simulink library "bcm"  (R2021b)
settings: Solver=VariableStepAuto  StartTime=0.0  StopTime=10.0  RelTol=1e-3
undefined symbols (not defined in the file or in its folder): ENUM_ANTITHEFT_ALARM, ENUM_ANTITHEFT_ARM, ENUM_ANTITHEFT_DISARM, ENUM_ANTITHEFT_WAIT, ENUM_GEARPOSNTOCAN_P, ENUM_PDKEYRAWLULOCK_INUNLOCK, ENUM_PDKEYRAWPS_INPS, ENUM_POWERSTA_ON, ENUM_POWERSTA_READY, ENUM_POWERSTA_STANDBY, ENUM_PWRSTASW_ON, ENUM_PWRSTASW_READY, ENUM_VEHICLETYPE_D21, ENUM_VEHICLETYPE_D31F25, ENUM_VEHICLETYPE_D31HAWD, ENUM_VEHICLETYPE_D31HRWD, ENUM_VEHICLETYPE_D31L24, FALSE, KBCM_ACCSwcPrsTmr_s, KBCM_ALMBrightnessDark_enum, KBCM_AmbBlue_enum, KBCM_AmbBreathT_ms, KBCM_AmbGreen_enum, KBCM_AmbMidPple_enum, KBCM_AmbRed_enum, KBCM_AmbTempCtrlEN_flg, KBCM_AmbTempT_s, KBCM_AmbWelModeENWait_s, KBCM_Antitheft_enum_ovrdflg, KBCM_Antitheft_enum_ovrdval, KBCM_APMDoorCtrlSta_flg_ovrdflg, KBCM_APMDoorCtrlSta_flg_ovrdval, KBCM_CmdKeepT_s, KBCM_CSWLightRstDebT_s, KBCM_CSWTurnLPRstT_s, KBCM_DelayTSW_flg, KBCM_DiagDRLOFF_flg, KBCM_DiagFLTC_mA, KBCM_DiagFMHT_s, KBCM_DiagFRTC_mA, KBCM_DiagRLTC_mA, KBCM_DiagRRTC_mA, KBCM_DrAPMRetryTimes_cnt, KBCM_DrOpenWdwOT_s, KBCM_DrOpenWdwReady_s, KBCM_ESSOffT_ms, KBCM_ESSOnT_ms, KBCM_FDCDKCReDetectT_K, KBCM_FDCDKCUSSFilterT_K, KBCM_HandleLampKeepT_s, KBCM_IVIRstHoldT_ms, KBCM_IVIRstTriggerT_ms, KBCM_ONDelayT_ms, KBCM_RAPSAbnFlashOFFT_ms, KBCM_RAPSAbnFlashONT_ms, KBCM_ReDetectT_K, KBCM_RightHandDriveEN_flg, KBCM_RLSLowSpdFilterT_s, KBCM_RmLampKeep_min, KBCM_RmLpKeyInT_s ... (+37)
libraries: simulink x389, $bdroot x11, hcu_lib x2
(part 6 of 13)

== system bcm/BCM/BCM/PTG/KeyDetected ==
  VBCM_PASDRMR_cm : Inport
  VBCM_USSFilterT_K : Inport  Port=2
  VBCM_PASDRML_cm : Inport  Port=3
  AND{,1,3..4} (4 alike) : Logic  AllPortsSameDT=off  OutDataTypeStr=boolean
  AND2 : Logic  Inputs=3  AllPortsSameDT=off  OutDataTypeStr=boolean
  AND5 : Logic  Inputs=3  AllPortsSameDT=off  OutDataTypeStr=boolean
  Add : Sum
  Add1 : Sum  Inputs=-++
  Add2 : Sum  Inputs=--
  CheckSignalAvailable : Subsystem
  Compare To Constant2 : simulink/Logic and Bit Operations/Compare To Constant  relop=<=  const=KBCM_SPTGUpperBound_cm  OutDataTypeStr=boolean
  Compare To Constant3 : simulink/Logic and Bit Operations/Compare To Constant  relop=>=  const=KBCM_SPTGLowerBound_cm  OutDataTypeStr=boolean
  Constant : Constant  Value=KBCM_SPTGRightBound_cm
  Constant10 : Constant  Value=KBCM_USSDis_cm
  Constant11 : Constant  Value=KBCM_SPTGUpperBoundOut_cm
  Constant12 : Constant  Value=KBCM_SPTGLowerBoundOut_cm
  Constant13 : Constant  Value=KBCM_SPTGRightBoundOut_cm
  Constant15 : Constant  Value=-1  OutDataTypeStr=single
  Constant16 : Constant  Value=0  OutDataTypeStr=single
  Constant17 : Constant  Value=KBCM_SPTGUpperBound_cm
  Constant18 : Constant  Value=KBCM_SPTGLowerBound_cm
  Constant2 : Constant  Value=KBCM_SPTGLeftBound_cm
  Constant3 : Constant  Value=-1  OutDataTypeStr=single
  Constant4 : Constant  Value=KBCM_USSDis_cm
  Constant5 : Constant  Value=0  OutDataTypeStr=single
  Constant6 : Constant  Value=KBCM_SPTGLeftBoundOut_cm
  Constant7 : Constant  Value=KBCM_USSDis_cm
  Constant8 : Constant  Value=KBCM_SPTGLeftBound_cm
  Constant9 : Constant  Value=KBCM_SPTGLeftBound_cm
  Data Type Conversion : DataTypeConversion  OutDataTypeStr=single
  Data Type Conversion1 : DataTypeConversion  OutDataTypeStr=single
  Data Type Conversion2 : DataTypeConversion  OutDataTypeStr=boolean
  Data Type Conversion3 : DataTypeConversion  OutDataTypeStr=boolean
  Detect Decrease : simulink/Logic and Bit Operations/Detect Decrease  vinit=0.0  OutDataTypeStr=boolean
  Detect Decrease1 : simulink/Logic and Bit Operations/Detect Decrease  vinit=0.0  OutDataTypeStr=boolean
  Equal : RelationalOperator  OutDataTypeStr=boolean  RndMeth=Simplest
  Gain : Gain  Gain=-1
  GreaterThan : RelationalOperator  Operator=<=  OutDataTypeStr=boolean  RndMeth=Simplest
  GreaterThan1 : RelationalOperator  Operator=<=  OutDataTypeStr=boolean  RndMeth=Simplest
  GreaterThan2 : RelationalOperator  OutDataTypeStr=boolean  RndMeth=Simplest
  Less Than : RelationalOperator  Operator=<=  OutDataTypeStr=boolean  RndMeth=Simplest
  Less Than1 : RelationalOperator  OutDataTypeStr=boolean  RndMeth=Simplest
  Product : Product
  Sum1 : Sum
  Sum2 : Sum  Inputs=|++
  Sum3 : Sum  Inputs=|+-
  Sum4 : Sum
  Switch{1..6} (6 alike) : Switch  Criteria=u2 > Threshold
  Target_h : Subsystem
  Unit Delay{1..6} (6 alike) : UnitDelay  SampleTime=-1  HasFrameUpgradeWarning=on
  cosRML : Subsystem
  KeyDetected : Outport
  KeyDetectedOut : Outport  Port=2
  wires:
  Constant4/1 -> CheckSignalAvailable/3(KBCM_USSDis_cm_IN)
  CheckSignalAvailable/1(VBCM_PASDRML_cm) -> cosRML/1(VBCM_PASDRML_cm), Target_h/1(VBCM_PASDRML_cm), Product/2
  CheckSignalAvailable/2(VBCM_PASDRMR_cm) -> Target_h/2(VBCM_PASDRMR_cm), cosRML/2(VBCM_PASDRMR_cm)
  CheckSignalAvailable/3(KBCM_USSDis_cm) -> Target_h/3(KBCM_USSDis_cm), cosRML/3(KBCM_USSDis_cm)
  Target_h/1(Target_h) -> Compare To Constant2/1, Compare To Constant3/1, Less Than/1, Less Than1/1
  Compare To Constant2/1 -> AND1/1
  Compare To Constant3/1 -> AND1/2
  AND1/1 -> AND2/2
  AND/1 -> AND2/1
  cosRML/1(cosRML) -> Product/1
  CheckSignalAvailable/4(CheckResult) -> [CheckResult]
  [CheckResult] -> AND2/3
  Detect Decrease/1 -> Switch2/2
  Switch2/1 -> Data Type Conversion/1
  Sum1/1 -> Switch2/3
  Unit Delay2/1 -> Switch3/2, Sum1/2, Switch4/2
  Constant3/1 -> Switch3/1
  Constant5/1 -> Switch3/3
  Switch3/1 -> Sum1/1
  Switch4/1 -> Data Type Conversion2/1, KeyDetected/1
  Unit Delay4/1 -> Switch4/1
  VBCM_PASDRML_cm/1 -> CheckSignalAvailable/1(VBCM_PASDRML_cm_IN)
  VBCM_PASDRMR_cm/1 -> CheckSignalAvailable/2(VBCM_PASDRMR_cm_IN)
  AND2/1 -> Unit Delay6/1, Detect Decrease/1
  GreaterThan1/1 -> AND4/1
  Add1/1 -> GreaterThan1/2
  [Target_x] -> GreaterThan1/1, GreaterThan2/1
  Product/1 -> [Target_x]
  [Target_x] -> Equal/1, GreaterThan/1
  Constant17/1 -> Sum2/1
  Constant11/1 -> Sum2/2
  Constant12/1 -> Sum3/2
  Constant18/1 -> Sum3/1
  [CheckResult] -> AND5/3
  AND3/1 -> AND5/1
  AND4/1 -> AND5/2
  AND5/1 -> Unit Delay1/1, Detect Decrease1/1
  Unit Delay5/1 -> Switch6/1
  Switch6/1 -> KeyDetectedOut/1, Data Type Conversion3/1
  Switch5/1 -> Sum4/1
  Constant16/1 -> Switch5/3
  Constant15/1 -> Switch5/1
  Unit Delay3/1 -> Switch6/2, Sum4/2, Switch5/2
  Sum4/1 -> Switch1/3
  Switch1/1 -> Data Type Conversion1/1
  Detect Decrease1/1 -> Switch1/2
  Sum2/1 -> Less Than/2
  Less Than/1 -> AND3/1
  Sum3/1 -> Less Than1/2
  Less Than1/1 -> AND3/2
  Constant10/1 -> Add1/2
  Constant9/1 -> Add1/1
  Constant13/1 -> Add1/3
  Constant7/1 -> Add/2
  Equal/1 -> AND/1
  GreaterThan/1 -> AND/2
  Constant/1 -> Add/1
  Add/1 -> GreaterThan/2
  GreaterThan2/1 -> AND4/2
  Constant2/1 -> Add2/1
  Constant6/1 -> Add2/2
  Add2/1 -> GreaterThan2/2
  Unit Delay1/1 -> Switch6/3
  Unit Delay6/1 -> Switch4/3
  Constant8/1 -> Gain/1
  Gain/1 -> Equal/2
  Data Type Conversion/1 -> Unit Delay2/1
  Data Type Conversion1/1 -> Unit Delay3/1
  Data Type Conversion2/1 -> Unit Delay4/1
  Data Type Conversion3/1 -> Unit Delay5/1
  VBCM_USSFilterT_K/1 -> [VBCM_USSFilterT_K]
  [VBCM_USSFilterT_K] -> Switch2/1
  [VBCM_USSFilterT_K] -> Switch1/1

== system bcm/BCM/BCM/PTG/Subsystem1 ==
  VAPM_PASDRMR_cm : Inport
  Add4 : Sum
  Compare To Constant1 : simulink/Logic and Bit Operations/Compare To Constant  relop=~=  const=0  OutDataTypeStr=boolean
  Compare To Constant6 : simulink/Logic and Bit Operations/Compare To Constant  relop===  const=0  OutDataTypeStr=boolean
  Compare To Constant8 : simulink/Logic and Bit Operations/Compare To Constant  relop===  const=255  OutDataTypeStr=boolean
  Constant1 : Constant  Value=0  OutDataTypeStr=uint8
  Constant12 : Constant  OutDataTypeStr=uint8
  Constant13 : Constant  Value=0  OutDataTypeStr=uint8
  Constant2 : Constant  OutDataTypeStr=uint8
  Constant3 : Constant  Value=KBCM_SPTGTOut_K
  Constant4 : Constant  Value=255  OutDataTypeStr=uint8
  Constant5 : Constant  Value=KBCM_SPTGTOut_K
  Detect Change : simulink/Logic and Bit Operations/Detect Change  vinit=0  OutDataTypeStr=boolean
  Equal : RelationalOperator  OutDataTypeStr=boolean  RndMeth=Simplest
  Equal1 : RelationalOperator  Operator===  OutDataTypeStr=boolean  RndMeth=Simplest
  Equal2 : RelationalOperator  Operator=~=  OutDataTypeStr=boolean  RndMeth=Simplest
  Logical Operator : Logic  Inputs=3  AllPortsSameDT=off  OutDataTypeStr=boolean
  Logical Operator2 : Logic  Operator=OR  AllPortsSameDT=off  OutDataTypeStr=boolean
  Switch{2..3,8..9} (4 alike) : Switch  Criteria=u2 > Threshold
  Unit Delay2 : UnitDelay  SampleTime=-1  HasFrameUpgradeWarning=on
  Unit Delay6 : UnitDelay  SampleTime=-1  HasFrameUpgradeWarning=on
  PASDRMR : Outport
  wires:
  Equal1/1 -> Logical Operator2/2
  Switch9/1 -> Add4/1
  Constant5/1 -> Equal2/2, Equal1/1
  Unit Delay6/1 -> Equal/1, Add4/2
  Compare To Constant8/1 -> Switch8/2
  Equal2/1 -> Logical Operator2/1
  Constant4/1 -> Switch3/3
  Switch2/1 -> Unit Delay2/1, Switch3/1
  Compare To Constant1/1 -> Logical Operator/2
  Logical Operator/1 -> Switch2/2
  Constant13/1 -> Switch9/1
  Add4/1 -> Switch8/1
  Unit Delay2/1 -> Switch2/3
  Constant12/1 -> Switch9/3
  Equal/1 -> Switch9/2
  Constant3/1 -> Equal/2
  Detect Change/1 -> Logical Operator/1
  Compare To Constant6/1 -> Logical Operator/3
  Constant1/1 -> Switch8/3
  Switch3/1 -> PASDRMR/1
  VAPM_PASDRMR_cm/1 -> Switch2/1, Detect Change/1, Compare To Constant1/1, Compare To Constant8/1
  Logical Operator2/1 -> Switch3/2
  Constant2/1 -> Equal1/2
  Switch8/1 -> Unit Delay6/1, Compare To Constant6/1, Equal2/1

== system bcm/BCM/BCM/PTG/Subsystem3 ==
  VAPM_PASDRML_cm : Inport
  Add4 : Sum
  Compare To Constant1 : simulink/Logic and Bit Operations/Compare To Constant  relop=~=  const=0  OutDataTypeStr=boolean
  Compare To Constant6 : simulink/Logic and Bit Operations/Compare To Constant  relop===  const=0  OutDataTypeStr=boolean
  Compare To Constant8 : simulink/Logic and Bit Operations/Compare To Constant  relop===  const=255  OutDataTypeStr=boolean
  Constant1 : Constant  Value=0  OutDataTypeStr=uint8
  Constant12 : Constant  OutDataTypeStr=uint8
  Constant13 : Constant  Value=0  OutDataTypeStr=uint8
  Constant2 : Constant  Value=0  OutDataTypeStr=uint8
  Constant3 : Constant  Value=KBCM_SPTGTOut_K
  Constant4 : Constant  Value=255  OutDataTypeStr=uint8
  Constant5 : Constant  Value=KBCM_SPTGTOut_K
  Detect Change : simulink/Logic and Bit Operations/Detect Change  vinit=0  OutDataTypeStr=boolean
  Equal : RelationalOperator  OutDataTypeStr=boolean  RndMeth=Simplest
  Equal1 : RelationalOperator  Operator===  OutDataTypeStr=boolean  RndMeth=Simplest
  Equal2 : RelationalOperator  Operator=~=  OutDataTypeStr=boolean  RndMeth=Simplest
  Logical Operator : Logic  Inputs=3  AllPortsSameDT=off  OutDataTypeStr=boolean
  Logical Operator2 : Logic  Operator=OR  AllPortsSameDT=off  OutDataTypeStr=boolean
  Switch{2..3,8..9} (4 alike) : Switch  Criteria=u2 > Threshold
  Unit Delay2 : UnitDelay  SampleTime=-1  HasFrameUpgradeWarning=on
  Unit Delay6 : UnitDelay  SampleTime=-1  HasFrameUpgradeWarning=on
  PASDRML : Outport
  wires:
  Constant2/1 -> Equal1/2
  Logical Operator2/1 -> Switch3/2
  VAPM_PASDRML_cm/1 -> Switch2/1, Detect Change/1, Compare To Constant1/1, Compare To Constant8/1
  Switch3/1 -> PASDRML/1
  Constant1/1 -> Switch8/3
  Compare To Constant6/1 -> Logical Operator/3
  Detect Change/1 -> Logical Operator/1
  Constant3/1 -> Equal/2
  Equal/1 -> Switch9/2
  Constant12/1 -> Switch9/3
  Unit Delay2/1 -> Switch2/3
  Add4/1 -> Switch8/1
  Constant13/1 -> Switch9/1
  Switch8/1 -> Equal2/1, Compare To Constant6/1, Unit Delay6/1
  Logical Operator/1 -> Switch2/2
  Compare To Constant1/1 -> Logical Operator/2
  Switch2/1 -> Unit Delay2/1, Switch3/1
  Constant4/1 -> Switch3/3
  Equal2/1 -> Logical Operator2/1
  Compare To Constant8/1 -> Switch8/2
  Unit Delay6/1 -> Equal/1, Add4/2
  Constant5/1 -> Equal2/2, Equal1/1
  Switch9/1 -> Add4/1
  Equal1/1 -> Logical Operator2/2

== system bcm/BCM/BCM/Personal_Setting/ACC ==
  UserNow : Inport
  Loadbar : Inport  Port=2
  UpdateReq : Inport  Port=3
  task_time_s : Inport  Port=4
  VINP_TimeGapLevel_enum : Inport  Port=5
  VINP_FlashACCLevelSta12_enum : Inport  Port=6
  VINP_FlashACCLevelSta34_enum : Inport  Port=7
  VINP_FlashACCLevelSta57_enum : Inport  Port=8
  VINP_SWC2LRightSta_flg : Inport  Port=9
  VINP_SWC2LLeftSta_flg : Inport  Port=10
  VINP_FDCVMCSpdCtrlModeSta_enum : Inport  Port=11
  VINP_ADASACCSta_enum : Inport  Port=12
  VINP_VehicleType_enum : Inport  Port=13
  AND : Logic  Inputs=3  AllPortsSameDT=off  OutDataTypeStr=boolean
  AND1 : Logic  AllPortsSameDT=off  OutDataTypeStr=boolean
  AND2 : Logic  AllPortsSameDT=off  OutDataTypeStr=boolean
  AND3 : Logic  AllPortsSameDT=off  OutDataTypeStr=boolean
  Chart : Stateflow chart  TreatAsAtomicUnit=on
  Compare To Constant : simulink/Logic and Bit Operations/Compare To Constant  relop===  const=1  OutDataTypeStr=boolean
  Compare To Constant1 : simulink/Logic and Bit Operations/Compare To Constant  relop=~=  const=0  OutDataTypeStr=boolean
  Compare To Constant2 : simulink/Logic and Bit Operations/Compare To Constant  relop=~=  const=5  OutDataTypeStr=boolean
  Compare To Constant3 : simulink/Logic and Bit Operations/Compare To Constant  relop=~=  const=6  OutDataTypeStr=boolean
  Constant : Constant  Value=4
  Constant1 : Constant  Value=KBCM_ACCSwcPrsTmr_s
  Constant3 : Constant  Value=KBCM_WaitACCChange_s
  Constant4 : Constant  Value=ENUM_VEHICLETYPE_D31L24
  Constant5 : Constant  Value=ENUM_VEHICLETYPE_D21
  Constant6 : Constant  Value=TRUE
  Constant7 : Constant  Value=FALSE
  Data Type Conversion : DataTypeConversion  OutDataTypeStr=uint8
  Divide : Product  Inputs=*/
  Divide1 : Product  Inputs=*/
  Equal : RelationalOperator  Operator===  OutDataTypeStr=boolean  RndMeth=Simplest
  Equal1 : RelationalOperator  Operator===  OutDataTypeStr=boolean  RndMeth=Simplest
  Logical Operator : Logic  Operator=OR  AllPortsSameDT=off  OutDataTypeStr=boolean
  Switch : Switch  Criteria=u2 ~= 0
  Switch1 : Switch  Criteria=u2 ~= 0
  Switch2 : Switch  Criteria=u2 ~= 0
  Switch3 : Switch  Criteria=u2 > Threshold
  VALUE_TYPE_ACC : Subsystem
  VBCM_TimeGapLevelSta_enum : Outport
  VBCM_ACCLevelMem12_enum : Outport  Port=2
  VBCM_ACCLevelMem34_enum : Outport  Port=3
  VBCM_ACCLevelMem57_enum : Outport  Port=4
  VBCM_LRightStaCmd_flg : Outport  Port=5
  VBCM_LLeftStaCmd_flg : Outport  Port=6
  wires:
  [task_time_s] -> Divide1/2
  Divide1/1 -> Chart/7(KBCM_WaitACCChange_s)
  Constant3/1 -> Divide1/1
  [task_time_s] -> Divide/2
  task_time_s/1 -> [task_time_s]
  Chart/2(VBCM_LLeftStaCmd_flg) -> Switch1/1
  Chart/1(VBCM_LRightStaCmd_flg) -> Switch/1
  [VINP_TimeGapLevel_enum] -> Switch2/3
  [VINP_TimeGapLevel_enum] -> Chart/2(VINP_TimeGapLevel_enum)
  VINP_TimeGapLevel_enum/1 -> [VINP_TimeGapLevel_enum]
  VALUE_TYPE_ACC/1(Setting) -> Switch2/1  "VBCM_TimeGapLevelSta_enum"
  Switch2/1 -> VBCM_TimeGapLevelSta_enum/1, [VBCM_TimeGapLevelSta_enum]  "VBCM_TimeGapLevelSta_enum"
  [VBCM_ACCUserSettingEN_flg] -> Switch2/2
  Switch1/1 -> VBCM_LLeftStaCmd_flg/1  "VBCM_LLeftStaCmd_flg"
  [VINP_SWC2LLeftSta_flg] -> Switch1/3
  [VBCM_ACCUserSettingEN_flg] -> Switch1/2
  [VINP_SWC2LRightSta_flg] -> Switch/3
  Switch/1 -> VBCM_LRightStaCmd_flg/1  "VBCM_LRightStaCmd_flg"
  [VBCM_ACCUserSettingEN_flg] -> Switch/2
  [VINP_SWC2LLeftSta_flg] -> Chart/5(VINP_SWC2LLeftSta_flg)
  [VINP_SWC2LRightSta_flg] -> Chart/4(VINP_SWC2LRightSta_flg)
  [VINP_SWC2LLeftSta_flg] -> AND3/2
  [VINP_SWC2LRightSta_flg] -> AND2/2
  VINP_SWC2LLeftSta_flg/1 -> [VINP_SWC2LLeftSta_flg]
  VINP_SWC2LRightSta_flg/1 -> [VINP_SWC2LRightSta_flg]
  Constant1/1 -> Divide/1
  Divide/1 -> Chart/6(KBCM_ACCSwcPrsTmr_s)
  [VBCM_TimeGapLevelSta_enum] -> Chart/3(VBCM_TimeGapLevelSta_enum)
  [UserNow] -> VALUE_TYPE_ACC/1(UserNow)
  UserNow/1 -> [UserNow]
  [VBCM_ACCChangeEnable_flg] -> Chart/1(VBCM_ACCChangeEnable_flg)
  [VBCM_ACCChangeEnable_flg] -> AND3/1
  [VBCM_ACCChangeEnable_flg] -> AND2/1
  AND3/1 -> VALUE_TYPE_ACC/5(MinusCmd)
  AND2/1 -> VALUE_TYPE_ACC/4(PlusCmd)
  AND1/1 -> [VBCM_ACCChangeEnable_flg]
  AND/1 -> AND1/2
  Compare To Constant/1 -> AND1/1
  VINP_ADASACCSta_enum/1 -> Compare To Constant1/1, Compare To Constant2/1, Compare To Constant3/1
  Compare To Constant3/1 -> AND/3
  Compare To Constant2/1 -> AND/2
  Compare To Constant1/1 -> AND/1
  VINP_FDCVMCSpdCtrlModeSta_enum/1 -> Compare To Constant/1
  VINP_FlashACCLevelSta12_enum/1 -> VALUE_TYPE_ACC/6(EEP_Set12)
  VINP_FlashACCLevelSta34_enum/1 -> VALUE_TYPE_ACC/7(EEP_Set34)
  VINP_FlashACCLevelSta57_enum/1 -> VALUE_TYPE_ACC/8(EEP_Set57)
  VALUE_TYPE_ACC/2(Set12) -> VBCM_ACCLevelMem12_enum/1  "VBCM_ACCLevelMem12_enum"
  VALUE_TYPE_ACC/3(Set34) -> VBCM_ACCLevelMem34_enum/1  "VBCM_ACCLevelMem34_enum"
  VALUE_TYPE_ACC/4(Set57) -> VBCM_ACCLevelMem57_enum/1  "VBCM_ACCLevelMem57_enum"
  Loadbar/1 -> VALUE_TYPE_ACC/2(Loadbar)
  UpdateReq/1 -> VALUE_TYPE_ACC/3(UpdateReq)
  Constant/1 -> Data Type Conversion/1
  Data Type Conversion/1 -> VALUE_TYPE_ACC/9(Default)
  VINP_VehicleType_enum/1 -> [VINP_VehicleType_enum]
  [VINP_VehicleType_enum] -> Equal/1
  Constant4/1 -> Equal/2
  Constant5/1 -> Equal1/2
  [VINP_VehicleType_enum] -> Equal1/1
  Equal/1 -> Logical Operator/1
  Equal1/1 -> Logical Operator/2
  Logical Operator/1 -> Switch3/2
  Constant7/1 -> Switch3/1
  Constant6/1 -> Switch3/3
  Switch3/1 -> [VBCM_ACCUserSettingEN_flg]

== system bcm/BCM/BCM/Personal_Setting/AmbLight ==
  UserNow : Inport
  Loadbar : Inport  Port=2
  VINP_CANMsgValidIVI1_flg : Inport  Port=3
  VINP_AmbLightSW_flg : Inport  Port=4
  VINP_FlashAmbFunEN_enum : Inport  Port=5
  VINP_AmbLightWlcmLightSW_flg : Inport  Port=6
  VINP_FlashAmbWelEN_enum : Inport  Port=7
  VINP_AmbLightDimInDarkSW_flg : Inport  Port=8
  VINP_FlashAmbDimEN_enum : Inport  Port=9
  VINP_LINKtoDRIVE_flg : Inport  Port=10
  VINP_FlashAmbLinkDriSta_enum : Inport  Port=11
  VINP_AmbLighLowBatAlertSW_flg : Inport  Port=12
  VINP_FlashAmbPwrWarnEN_enum : Inport  Port=13
  VINP_AmbLighSafetyAlertSW_flg : Inport  Port=14
  VINP_FlashAmbODAEN_enum : Inport  Port=15
  VINP_AmbLightColorSet_enum : Inport  Port=16
  VINP_FlashAmbColorSta1_enum : Inport  Port=17
  VINP_FlashAmbColorSta2_enum : Inport  Port=18
  VINP_FlashAmbColorSta3_enum : Inport  Port=19
  VINP_FlashAmbColorSta4_enum : Inport  Port=20
  VINP_FlashAmbColorSta5_enum : Inport  Port=21
  VINP_FlashAmbColorSta7_enum : Inport  Port=22
  VINP_AmbLightBrightnessSet_enum : Inport  Port=23
  VINP_FlashAmbBrightnessSta1_enum : Inport  Port=24
  VINP_FlashAmbBrightnessSta2_enum : Inport  Port=25
  VINP_FlashAmbBrightnessSta3_enum : Inport  Port=26
  VINP_FlashAmbBrightnessSta4_enum : Inport  Port=27
  VINP_FlashAmbBrightnessSta5_enum : Inport  Port=28
  VINP_FlashAmbBrightnessSta7_enum : Inport  Port=29
  Constant{,3..7} (6 alike) : Constant  OutDataTypeStr=boolean
  Constant1 : Constant  Value=28  OutDataTypeStr=uint8
  Constant10 : Constant  Value=101  OutDataTypeStr=uint8
  Constant2 : Constant  Value=50  OutDataTypeStr=uint8
  Constant9 : Constant  Value=64  OutDataTypeStr=uint8
  Data Type Conversion : DataTypeConversion  OutDataTypeStr=uint8
  Ground : Ground
  TOGGLE_TYPE_AmbDimEN : Subsystem
  TOGGLE_TYPE_AmbFunEN : Subsystem
  TOGGLE_TYPE_AmbLinkDriSta : Subsystem
  TOGGLE_TYPE_AmbODAEN : Subsystem
  TOGGLE_TYPE_AmbPwrWarnEN : Subsystem
  TOGGLE_TYPE_AmbWelEN : Subsystem
  VALUE_TYPE_AmbBrightnessSta : Subsystem
  VALUE_TYPE_AmbColorSta : Subsystem
  VBCM_UserNow_enum : Outport
  FDC_BCM_AmbFunEN_Sta : Outport  Port=2
  VBCM_AmbFunENMem_enum : Outport  Port=3
  FDC_BCM_AmbWelEN_Sta : Outport  Port=4
  VBCM_AmbWelENMem_enum : Outport  Port=5
  FDC_BCM_AmbDimEN_Sta : Outport  Port=6
  VBCM_AmbDimENMem_enum : Outport  Port=7
  FDC_BCM_AmbLinkDriSta_Sta : Outport  Port=8
  VBCM_AmbLinkDriStaMem_enum : Outport  Port=9
  FDC_BCM_AmbPwrWarnEN_Sta : Outport  Port=10
  VBCM_AmbPwrWarnENMem_enum : Outport  Port=11
  FDC_BCM_AmbODAEN_Sta : Outport  Port=12
  VBCM_AmbODAENMem_enum : Outport  Port=13
  FDC_BCM_AmbColorSta_Sta : Outport  Port=14
  VBCM_AmbColorSta1_enum : Outport  Port=15
  VBCM_AmbColorSta2_enum : Outport  Port=16
  VBCM_AmbColorSta3_enum : Outport  Port=17
  VBCM_AmbColorSta4_enum : Outport  Port=18
  VBCM_AmbColorSta5_enum : Outport  Port=19
  VBCM_AmbColorSta7_enum : Outport  Port=20
  FDC_BCM_AmbBrightSta_Sta : Outport  Port=21  OutDataTypeStr=uint8
  VBCM_AmbBrightnessSta1_enum : Outport  Port=22  OutDataTypeStr=uint8
  VBCM_AmbBrightnessSta2_enum : Outport  Port=23
  VBCM_AmbBrightnessSta3_enum : Outport  Port=24
  VBCM_AmbBrightnessSta4_enum : Outport  Port=25
  VBCM_AmbBrightnessSta5_enum : Outport  Port=26
  VBCM_AmbBrightnessSta7_enum : Outport  Port=27
  wires:
  VALUE_TYPE_AmbBrightnessSta/3(Set2) -> VBCM_AmbBrightnessSta2_enum/1
  VALUE_TYPE_AmbBrightnessSta/2(Set1) -> VBCM_AmbBrightnessSta1_enum/1
  [UserNow] -> VALUE_TYPE_AmbBrightnessSta/1(UserNow)
  VALUE_TYPE_AmbBrightnessSta/1(Setting) -> FDC_BCM_AmbBrightSta_Sta/1
  TOGGLE_TYPE_AmbFunEN/1(Setting) -> FDC_BCM_AmbFunEN_Sta/1
  [Loadbar] -> VALUE_TYPE_AmbColorSta/2(Loadbar)
  VALUE_TYPE_AmbBrightnessSta/6(Set5) -> VBCM_AmbBrightnessSta5_enum/1
  TOGGLE_TYPE_AmbFunEN/2(Set) -> VBCM_AmbFunENMem_enum/1
  VALUE_TYPE_AmbBrightnessSta/7(Set7) -> VBCM_AmbBrightnessSta7_enum/1
  VALUE_TYPE_AmbBrightnessSta/4(Set3) -> VBCM_AmbBrightnessSta3_enum/1
  [UserNow] -> VALUE_TYPE_AmbColorSta/1(UserNow)
  VALUE_TYPE_AmbBrightnessSta/5(Set4) -> VBCM_AmbBrightnessSta4_enum/1
  [Loadbar] -> VALUE_TYPE_AmbBrightnessSta/2(Loadbar)
  UserNow/1 -> [UserNow]
  Loadbar/1 -> [Loadbar]
  VALUE_TYPE_AmbColorSta/1(Setting) -> FDC_BCM_AmbColorSta_Sta/1
  VALUE_TYPE_AmbColorSta/2(Set1) -> VBCM_AmbColorSta1_enum/1
  VALUE_TYPE_AmbColorSta/3(Set2) -> VBCM_AmbColorSta2_enum/1
  VALUE_TYPE_AmbColorSta/4(Set3) -> VBCM_AmbColorSta3_enum/1
  VALUE_TYPE_AmbColorSta/5(Set4) -> VBCM_AmbColorSta4_enum/1
  VALUE_TYPE_AmbColorSta/6(Set5) -> VBCM_AmbColorSta5_enum/1
  VALUE_TYPE_AmbColorSta/7(Set7) -> VBCM_AmbColorSta7_enum/1
  [UserNow] -> TOGGLE_TYPE_AmbFunEN/1(UserNow)
  [Loadbar] -> TOGGLE_TYPE_AmbFunEN/2(Loadbar)
  VINP_AmbLightSW_flg/1 -> TOGGLE_TYPE_AmbFunEN/3(iviCMD)
  VINP_FlashAmbFunEN_enum/1 -> TOGGLE_TYPE_AmbFunEN/4(EEP_Set)
  Constant/1 -> TOGGLE_TYPE_AmbFunEN/5(Default)
  Constant9/1 -> VALUE_TYPE_AmbColorSta/11(NoReqV)
  Constant1/1 -> VALUE_TYPE_AmbColorSta/12(Default)
  VINP_FlashAmbColorSta7_enum/1 -> VALUE_TYPE_AmbColorSta/9(EEP_Set7)
  VINP_FlashAmbColorSta5_enum/1 -> VALUE_TYPE_AmbColorSta/8(EEP_Set5)
  VINP_FlashAmbColorSta4_enum/1 -> VALUE_TYPE_AmbColorSta/7(EEP_Set4)
  VINP_FlashAmbColorSta3_enum/1 -> VALUE_TYPE_AmbColorSta/6(EEP_Set3)
  VINP_FlashAmbColorSta2_enum/1 -> VALUE_TYPE_AmbColorSta/5(EEP_Set2)
  VINP_FlashAmbColorSta1_enum/1 -> VALUE_TYPE_AmbColorSta/4(EEP_Set1)
  Constant10/1 -> VALUE_TYPE_AmbBrightnessSta/11(NoReqV)
  Constant2/1 -> VALUE_TYPE_AmbBrightnessSta/12(Default)
  VINP_FlashAmbBrightnessSta7_enum/1 -> VALUE_TYPE_AmbBrightnessSta/9(EEP_Set7)
  VINP_FlashAmbBrightnessSta5_enum/1 -> VALUE_TYPE_AmbBrightnessSta/8(EEP_Set5)
  VINP_FlashAmbBrightnessSta4_enum/1 -> VALUE_TYPE_AmbBrightnessSta/7(EEP_Set4)
  VINP_FlashAmbBrightnessSta3_enum/1 -> VALUE_TYPE_AmbBrightnessSta/6(EEP_Set3)
  VINP_FlashAmbBrightnessSta2_enum/1 -> VALUE_TYPE_AmbBrightnessSta/5(EEP_Set2)
  VINP_FlashAmbBrightnessSta1_enum/1 -> VALUE_TYPE_AmbBrightnessSta/4(EEP_Set1)
  VINP_AmbLightBrightnessSet_enum/1 -> VALUE_TYPE_AmbBrightnessSta/3(iviCMD)
  [UserNow] -> TOGGLE_TYPE_AmbWelEN/1(UserNow)
  [Loadbar] -> TOGGLE_TYPE_AmbWelEN/2(Loadbar)
  Constant3/1 -> TOGGLE_TYPE_AmbWelEN/5(Default)
  VINP_AmbLightWlcmLightSW_flg/1 -> TOGGLE_TYPE_AmbWelEN/3(iviCMD)
  VINP_FlashAmbWelEN_enum/1 -> TOGGLE_TYPE_AmbWelEN/4(EEP_Set)
  TOGGLE_TYPE_AmbWelEN/1(Setting) -> FDC_BCM_AmbWelEN_Sta/1
  TOGGLE_TYPE_AmbWelEN/2(Set) -> VBCM_AmbWelENMem_enum/1
  [UserNow] -> TOGGLE_TYPE_AmbDimEN/1(UserNow)
  Constant4/1 -> TOGGLE_TYPE_AmbDimEN/5(Default)
  [Loadbar] -> TOGGLE_TYPE_AmbDimEN/2(Loadbar)
  VINP_AmbLightDimInDarkSW_flg/1 -> TOGGLE_TYPE_AmbDimEN/3(iviCMD)
  VINP_FlashAmbDimEN_enum/1 -> TOGGLE_TYPE_AmbDimEN/4(EEP_Set)
  TOGGLE_TYPE_AmbDimEN/1(Setting) -> FDC_BCM_AmbDimEN_Sta/1
  TOGGLE_TYPE_AmbDimEN/2(Set) -> VBCM_AmbDimENMem_enum/1
  [UserNow] -> TOGGLE_TYPE_AmbLinkDriSta/1(UserNow)
  Constant5/1 -> TOGGLE_TYPE_AmbLinkDriSta/8(Default)
  [Loadbar] -> TOGGLE_TYPE_AmbLinkDriSta/2(Loadbar)
  VINP_LINKtoDRIVE_flg/1 -> TOGGLE_TYPE_AmbLinkDriSta/6(iviCMD)
  VINP_FlashAmbLinkDriSta_enum/1 -> TOGGLE_TYPE_AmbLinkDriSta/7(EEP_Set)
  TOGGLE_TYPE_AmbLinkDriSta/1(Setting) -> FDC_BCM_AmbLinkDriSta_Sta/1
  TOGGLE_TYPE_AmbLinkDriSta/2(Set) -> VBCM_AmbLinkDriStaMem_enum/1
  Constant6/1 -> TOGGLE_TYPE_AmbPwrWarnEN/5(Default)
  [UserNow] -> TOGGLE_TYPE_AmbPwrWarnEN/1(UserNow)
  [Loadbar] -> TOGGLE_TYPE_AmbPwrWarnEN/2(Loadbar)
  VINP_AmbLighLowBatAlertSW_flg/1 -> TOGGLE_TYPE_AmbPwrWarnEN/3(iviCMD)
  VINP_FlashAmbPwrWarnEN_enum/1 -> TOGGLE_TYPE_AmbPwrWarnEN/4(EEP_Set)
  TOGGLE_TYPE_AmbPwrWarnEN/1(Setting) -> FDC_BCM_AmbPwrWarnEN_Sta/1
  TOGGLE_TYPE_AmbPwrWarnEN/2(Set) -> VBCM_AmbPwrWarnENMem_enum/1
  [UserNow] -> TOGGLE_TYPE_AmbODAEN/1(UserNow)
  [Loadbar] -> TOGGLE_TYPE_AmbODAEN/2(Loadbar)
  Constant7/1 -> TOGGLE_TYPE_AmbODAEN/5(Default)
  VINP_AmbLighSafetyAlertSW_flg/1 -> TOGGLE_TYPE_AmbODAEN/3(iviCMD)
  VINP_FlashAmbODAEN_enum/1 -> TOGGLE_TYPE_AmbODAEN/4(EEP_Set)
  TOGGLE_TYPE_AmbODAEN/1(Setting) -> FDC_BCM_AmbODAEN_Sta/1
  TOGGLE_TYPE_AmbODAEN/2(Set) -> VBCM_AmbODAENMem_enum/1
  VINP_CANMsgValidIVI1_flg/1 -> [VINP_CANMsgValidIVI1_flg]
  [VINP_CANMsgValidIVI1_flg] -> VALUE_TYPE_AmbColorSta/10(VINP_CANMsgValidIVI1_flg)
  [VINP_CANMsgValidIVI1_flg] -> VALUE_TYPE_AmbBrightnessSta/10(VINP_CANMsgValidIVI1_flg)
  [UserNow] -> Data Type Conversion/1
  Data Type Conversion/1 -> VBCM_UserNow_enum/1
  VINP_AmbLightColorSet_enum/1 -> [VINP_AmbLightColorSet_enum]
  [VINP_AmbLightColorSet_enum] -> VALUE_TYPE_AmbColorSta/3(iviCMD)
  Ground/1 -> TOGGLE_TYPE_AmbLinkDriSta/3(UpdateReq)
  [VINP_AmbLightColorSet_enum] -> TOGGLE_TYPE_AmbLinkDriSta/5(VINP_AmbLightColorSet_enum)
  [VINP_CANMsgValidIVI1_flg] -> TOGGLE_TYPE_AmbLinkDriSta/4(VINP_CANMsgValidIVI1_flg)

== system bcm/BCM/BCM/Personal_Setting/Autolock ==
  UserNow : Inport
  Loadbar : Inport  Port=2
  VBCM_SettingUpdateReq_enum : Inport  Port=3
  VINP_IVIStoppingUnlockSWSta_flg : Inport  Port=4
  VINP_FlashAutoLock_enum : Inport  Port=5
  VINP_IVIDrivingLockSWSta_flg : Inport  Port=6
  VINP_FlashAutoUnlock_enum : Inport  Port=7
  VINP_VehicleType_enum : Inport  Port=8
  Constant : Constant  Value=TRUE
  Constant1 : Constant  Value=TRUE
  Constant2 : Constant  Value=ENUM_VEHICLETYPE_D31L24
  Constant4 : Constant  Value=TRUE
  Constant5 : Constant  Value=FALSE
  Constant8 : Constant  Value=FALSE
  Constant9 : Constant  Value=FALSE
  Equal : RelationalOperator  Operator===  OutDataTypeStr=boolean  RndMeth=Simplest
  Switch : Switch  Criteria=u2 > Threshold
  Switch1 : Switch  Criteria=u2 ~= 0
  Switch3 : Switch  Criteria=u2 ~= 0
  TOGGLE_TYPE_AutoLock : Subsystem
  TOGGLE_TYPE_AutoUnlock : Subsystem
  VBCM_AutoLockSta_flg : Outport
  VBCM_AutoLockMem_enum : Outport  Port=2
  VBCM_AutoUnlockSta_flg : Outport  Port=3
  VBCM_AutoUnlockMem_enum : Outport  Port=4
  wires:
  [VBCM_SpeedLockFunEN] -> Switch1/2
  TOGGLE_TYPE_AutoUnlock/1(Setting) -> Switch1/1  "VBCM_AutoUnlockSta_flg"
  Constant9/1 -> Switch1/3
  Switch1/1 -> VBCM_AutoUnlockSta_flg/1
  Switch3/1 -> VBCM_AutoLockSta_flg/1
  Constant8/1 -> Switch3/3
  TOGGLE_TYPE_AutoLock/1(Setting) -> Switch3/1  "VBCM_AutoLockSta_flg"
  [VBCM_SpeedLockFunEN] -> Switch3/2
  VINP_FlashAutoUnlock_enum/1 -> TOGGLE_TYPE_AutoUnlock/5(EEP_Set)
  VINP_IVIStoppingUnlockSWSta_flg/1 -> TOGGLE_TYPE_AutoUnlock/4(iviCMD)
  VINP_FlashAutoLock_enum/1 -> TOGGLE_TYPE_AutoLock/5(EEP_Set)
  VINP_IVIDrivingLockSWSta_flg/1 -> TOGGLE_TYPE_AutoLock/4(iviCMD)
  TOGGLE_TYPE_AutoUnlock/2(Set) -> VBCM_AutoUnlockMem_enum/1
  TOGGLE_TYPE_AutoLock/2(Set) -> VBCM_AutoLockMem_enum/1
  Constant1/1 -> TOGGLE_TYPE_AutoUnlock/6(Default)
  Constant/1 -> TOGGLE_TYPE_AutoLock/6(Default)
  [VBCM_SettingUpdateReq_enum] -> TOGGLE_TYPE_AutoUnlock/3(UpdateReq)
  [UserNow] -> TOGGLE_TYPE_AutoUnlock/1(UserNow)
  [Loadbar] -> TOGGLE_TYPE_AutoUnlock/2(Loadbar)
  [VBCM_SettingUpdateReq_enum] -> TOGGLE_TYPE_AutoLock/3(UpdateReq)
  [Loadbar] -> TOGGLE_TYPE_AutoLock/2(Loadbar)
  [UserNow] -> TOGGLE_TYPE_AutoLock/1(UserNow)
  VBCM_SettingUpdateReq_enum/1 -> [VBCM_SettingUpdateReq_enum]
  Loadbar/1 -> [Loadbar]
  UserNow/1 -> [UserNow]
  VINP_VehicleType_enum/1 -> [VINP_VehicleType_enum]
  [VINP_VehicleType_enum] -> Equal/1
  Constant2/1 -> Equal/2
  Equal/1 -> Switch/2
  Constant5/1 -> Switch/1
  Constant4/1 -> Switch/3
  Switch/1 -> [VBCM_SpeedLockFunEN]

== system bcm/BCM/BCM/Personal_Setting/DKC_Lock_Setting ==
  UserNow : Inport
  Loadbar : Inport  Port=2
  VINP_ApproachUnlockSW_flg : Inport  Port=3
  VINP_FlashWalkInUnLkEn_enum : Inport  Port=4
  VINP_IVICarWashModeCmd_flg : Inport  Port=5
  VINP_WalkawayLockSW_flg : Inport  Port=6
  VINP_FlashWalkOutLkEn_enum : Inport  Port=7
  Constant : Constant  OutDataTypeStr=boolean
  Constant1 : Constant  Value=FALSE
  Constant3 : Constant  OutDataTypeStr=boolean
  Switch : Switch  Criteria=u2 > Threshold
  TOGGLE_TYPE_WalkInUnlock : Subsystem
  TOGGLE_TYPE_WalkOutLock : Subsystem
  FDC_BCM_WalkInUnLkEnFun_Sta : Outport
  VBCM_WalkInUnLkEnMem_enum : Outport  Port=2
  FDC_BCM_WalkOutLkEnFun_Sta : Outport  Port=3
  VBCM_WalkOutLkEnMem_enum : Outport  Port=4
  wires:
  TOGGLE_TYPE_WalkOutLock/2(Set) -> VBCM_WalkOutLkEnMem_enum/1
  VINP_FlashWalkOutLkEn_enum/1 -> TOGGLE_TYPE_WalkOutLock/4(EEP_Set)
  VINP_WalkawayLockSW_flg/1 -> TOGGLE_TYPE_WalkOutLock/3(iviCMD)
  Constant3/1 -> TOGGLE_TYPE_WalkOutLock/5(Default)
  [Loadbar] -> TOGGLE_TYPE_WalkOutLock/2(Loadbar)
  [UserNow] -> TOGGLE_TYPE_WalkOutLock/1(UserNow)
  Constant/1 -> TOGGLE_TYPE_WalkInUnlock/5(Default)
  VINP_FlashWalkInUnLkEn_enum/1 -> TOGGLE_TYPE_WalkInUnlock/4(EEP_Set)
  VINP_ApproachUnlockSW_flg/1 -> TOGGLE_TYPE_WalkInUnlock/3(iviCMD)
  [Loadbar] -> TOGGLE_TYPE_WalkInUnlock/2(Loadbar)
  [UserNow] -> TOGGLE_TYPE_WalkInUnlock/1(UserNow)
  Loadbar/1 -> [Loadbar]
  UserNow/1 -> [UserNow]
  TOGGLE_TYPE_WalkInUnlock/2(Set) -> VBCM_WalkInUnLkEnMem_enum/1
  TOGGLE_TYPE_WalkInUnlock/1(Setting) -> FDC_BCM_WalkInUnLkEnFun_Sta/1
  VINP_IVICarWashModeCmd_flg/1 -> Switch/2
  TOGGLE_TYPE_WalkOutLock/1(Setting) -> Switch/3
  Switch/1 -> FDC_BCM_WalkOutLkEnFun_Sta/1
  Constant1/1 -> Switch/1

== system bcm/BCM/BCM/Personal_Setting/FlasherSignal ==
  UserNow : Inport
  Loadbar : Inport  Port=2
  VINP_TurnSwTimeSet_enum : Inport  Port=3
  VINP_FlashTurnSwTimeSetSta123_enum : Inport  Port=4
  VINP_FlashTurnSwTimeSetSta457_enum : Inport  Port=5
  VINP_CANMsgValidIVI2_flg : Inport  Port=6
  Constant : Constant  Value=3  OutDataTypeStr=uint8
  Constant1 : Constant  Value=0  OutDataTypeStr=uint8
  VALUE_TYPE_FlasherSignal : Subsystem
  FDC_BCM_TurnSwTSetSta_Sta : Outport
  VBCM_TurnSwTimeSetSta123_enum : Outport  Port=2
  VBCM_TurnSwTimeSetSta457_enum : Outport  Port=3
  wires:
  UserNow/1 -> VALUE_TYPE_FlasherSignal/1(UserNow)
  Loadbar/1 -> VALUE_TYPE_FlasherSignal/2(Loadbar)
  VINP_TurnSwTimeSet_enum/1 -> VALUE_TYPE_FlasherSignal/3(iviCMD)
  VINP_FlashTurnSwTimeSetSta123_enum/1 -> VALUE_TYPE_FlasherSignal/4(EEP_Set123)
  VINP_FlashTurnSwTimeSetSta457_enum/1 -> VALUE_TYPE_FlasherSignal/5(EEP_Set457)
  Constant/1 -> VALUE_TYPE_FlasherSignal/7(NoReqV)
  Constant1/1 -> VALUE_TYPE_FlasherSignal/8(Default)
  VALUE_TYPE_FlasherSignal/1(Setting) -> FDC_BCM_TurnSwTSetSta_Sta/1
  VALUE_TYPE_FlasherSignal/2(Set123) -> VBCM_TurnSwTimeSetSta123_enum/1
  VALUE_TYPE_FlasherSignal/3(Set457) -> VBCM_TurnSwTimeSetSta457_enum/1
  VINP_CANMsgValidIVI2_flg/1 -> VALUE_TYPE_FlasherSignal/6(VINP_CANMsgValidIVI2_flg)

== system bcm/BCM/BCM/Personal_Setting/FollowMeHome ==
  UserNow : Inport
  Loadbar : Inport  Port=2
  VINP_FollowMeSW_flg : Inport  Port=3
  VINP_FlashFollowMeENFun_enum : Inport  Port=4
  Constant : Constant  OutDataTypeStr=boolean
  LockSetting : Subsystem
  FDC_BCM_FollowMeENFun_Sta : Outport
  VBCM_FollowMeENMem_enum : Outport  Port=2
  wires:
  LockSetting/1(Setting) -> FDC_BCM_FollowMeENFun_Sta/1
  LockSetting/2(Set) -> VBCM_FollowMeENMem_enum/1
  UserNow/1 -> [UserNow]
  Loadbar/1 -> [Loadbar]
  [UserNow] -> LockSetting/1(UserNow)
  [Loadbar] -> LockSetting/2(Loadbar)
  VINP_FollowMeSW_flg/1 -> LockSetting/3(iviCMD)
  VINP_FlashFollowMeENFun_enum/1 -> LockSetting/4(EEP_Set)
  Constant/1 -> LockSetting/5(Default)

== system bcm/BCM/BCM/Personal_Setting/LockSetting ==
  UserNow : Inport
  Loadbar : Inport  Port=2
  VINP_SetUnlockSingle_flg : Inport  Port=3
  VINP_FlashLockSettingSta_enum : Inport  Port=4
  Constant : Constant  Value=0  OutDataTypeStr=boolean
  LockSetting : Subsystem
  VBCM_LockSetting_flg : Outport
  VBCM_LockSettingStaMem_enum : Outport  Port=2
  wires:
  Constant/1 -> LockSetting/5(Default)
  VINP_FlashLockSettingSta_enum/1 -> LockSetting/4(EEP_Set)
  VINP_SetUnlockSingle_flg/1 -> LockSetting/3(iviCMD)
  [Loadbar] -> LockSetting/2(Loadbar)
  [UserNow] -> LockSetting/1(UserNow)
  Loadbar/1 -> [Loadbar]
  UserNow/1 -> [UserNow]
  LockSetting/2(Set) -> VBCM_LockSettingStaMem_enum/1
  LockSetting/1(Setting) -> VBCM_LockSetting_flg/1

== system bcm/BCM/BCM/Personal_Setting/PTG ==
  note: Remove_After_Account_Switch_Function_Applied
  UserNow : Inport
  Loadbar : Inport  Port=2
  VINP_IVIPTGOpenHeight_enum : Inport  Port=3
  VINP_FlashPTGOpenHeight12_enum : Inport  Port=4
  VINP_FlashPTGOpenHeight34_enum : Inport  Port=5
  VINP_FlashPTGOpenHeight57_enum : Inport  Port=6
  VINP_PTGIsSetHeight_flg : Inport  Port=7
  VINP_BPPTGIsSetHeightSta_flg : Inport  Port=8
  VINP_PTGLeftHallPosn_cnt : Inport  Port=9
  VINP_FlashPTGUserHeight1_cnt : Inport  Port=10
  VINP_FlashPTGUserHeight2_cnt : Inport  Port=11
  VINP_FlashPTGUserHeight3_cnt : Inport  Port=12
  VINP_FlashPTGUserHeight4_cnt : Inport  Port=13
  VINP_FlashPTGUserHeight5_cnt : Inport  Port=14
  VINP_FlashPTGUserHeight7_cnt : Inport  Port=15
  VINP_CANMsgValidIVI2_flg : Inport  Port=16
  VINP_CANMsgValidBodyZonePS1_flg : Inport  Port=17
  VINP_LeftHallPos_cnt : Inport  Port=18
  VINP_VehicleType_enum : Inport  Port=19
  Compare To Constant : simulink/Logic and Bit Operations/Compare To Constant  relop=<=  const=0  OutDataTypeStr=boolean
  Compare To Constant1 : simulink/Logic and Bit Operations/Compare To Constant  relop=<=  const=0  OutDataTypeStr=boolean
  Compare To Constant2 : simulink/Logic and Bit Operations/Compare To Constant  relop=>=  const=1023  OutDataTypeStr=boolean
  Constant : Constant  Value=1023
  Constant10 : Constant  Value=ENUM_VEHICLETYPE_D21
  Constant11 : Constant  Value=680
  Constant12 : Constant  Value=520
  Constant6 : Constant  Value=5
  Constant7 : Constant  Value=ZERO_INT
  Constant9 : Constant  Value=1023
  Data Type Conversion{1,7..10,14} (6 alike) : DataTypeConversion  OutDataTypeStr=uint16
  Data Type Conversion6 : DataTypeConversion  OutDataTypeStr=uint8
  Equal : RelationalOperator  Operator===  OutDataTypeStr=boolean  RndMeth=Simplest
  OR : Logic  Operator=OR  AllPortsSameDT=off  OutDataTypeStr=boolean
  Switch{,1,3..4} (4 alike) : Switch  Criteria=u2 ~= 0
  Switch2 : Switch  Criteria=u2 > Threshold
  VALUE_TYPE_FlasherSignal : Subsystem
  VALUE_TYPE_PTGUserSetMaxHeight : Subsystem
  VBCM_PTGOpenHeightSta_enum : Outport
  VBCM_UserHeightSet_cnt : Outport  Port=2
  VBCM_PTGUserHeight1_cnt : Outport  Port=3
  VBCM_PTGUserHeight2_cnt : Outport  Port=4
  VBCM_PTGUserHeight3_cnt : Outport  Port=5
  VBCM_PTGUserHeight4_cnt : Outport  Port=6
  VBCM_PTGUserHeight5_cnt : Outport  Port=7
  VBCM_PTGUserHeight7_cnt : Outport  Port=8
  VBCM_PTGOpenHeight12_enum : Outport  Port=9
  VBCM_PTGOpenHeight34_enum : Outport  Port=10
  VBCM_PTGOpenHeight57_enum : Outport  Port=11
  wires:
  Data Type Conversion1/1 -> VALUE_TYPE_PTGUserSetMaxHeight/11(NoReqV)
  VINP_FlashPTGUserHeight7_cnt/1 -> VALUE_TYPE_PTGUserSetMaxHeight/10(EEP_Set7)
  VINP_FlashPTGUserHeight5_cnt/1 -> VALUE_TYPE_PTGUserSetMaxHeight/9(EEP_Set5)
  VINP_FlashPTGUserHeight4_cnt/1 -> VALUE_TYPE_PTGUserSetMaxHeight/8(EEP_Set4)
  VINP_FlashPTGUserHeight3_cnt/1 -> VALUE_TYPE_PTGUserSetMaxHeight/7(EEP_Set3)
  VINP_FlashPTGUserHeight2_cnt/1 -> VALUE_TYPE_PTGUserSetMaxHeight/6(EEP_Set2)
  VALUE_TYPE_PTGUserSetMaxHeight/7(Set7) -> VBCM_PTGUserHeight7_cnt/1
  VALUE_TYPE_PTGUserSetMaxHeight/6(Set5) -> VBCM_PTGUserHeight5_cnt/1
  VALUE_TYPE_PTGUserSetMaxHeight/5(Set4) -> VBCM_PTGUserHeight4_cnt/1
  VALUE_TYPE_PTGUserSetMaxHeight/4(Set3) -> VBCM_PTGUserHeight3_cnt/1
  VALUE_TYPE_PTGUserSetMaxHeight/3(Set2) -> VBCM_PTGUserHeight2_cnt/1
  VALUE_TYPE_PTGUserSetMaxHeight/2(Set1) -> VBCM_PTGUserHeight1_cnt/1
  VALUE_TYPE_PTGUserSetMaxHeight/1(Setting) -> VBCM_UserHeightSet_cnt/1
  Constant/1 -> Data Type Conversion1/1
  [Loadbar] -> VALUE_TYPE_PTGUserSetMaxHeight/2(Loadbar)
  [UserNow] -> VALUE_TYPE_PTGUserSetMaxHeight/1(UserNow)
  Loadbar/1 -> [Loadbar]
  UserNow/1 -> [UserNow]
  [UserNow] -> VALUE_TYPE_FlasherSignal/1(UserNow)
  [Loadbar] -> VALUE_TYPE_FlasherSignal/2(Loadbar)
  VINP_IVIPTGOpenHeight_enum/1 -> VALUE_TYPE_FlasherSignal/3(iviCMD)
  VALUE_TYPE_FlasherSignal/1(Setting) -> VBCM_PTGOpenHeightSta_enum/1
  Constant6/1 -> Data Type Conversion6/1
  Data Type Conversion6/1 -> VALUE_TYPE_FlasherSignal/8(NoReqV)
  VALUE_TYPE_FlasherSignal/2(Set12) -> VBCM_PTGOpenHeight12_enum/1
  VALUE_TYPE_FlasherSignal/3(Set34) -> VBCM_PTGOpenHeight34_enum/1
  VALUE_TYPE_FlasherSignal/4(Set57) -> VBCM_PTGOpenHeight57_enum/1
  VINP_FlashPTGOpenHeight34_enum/1 -> VALUE_TYPE_FlasherSignal/5(EEP_Set34)
  VINP_FlashPTGOpenHeight57_enum/1 -> VALUE_TYPE_FlasherSignal/6(EEP_Set57)
  VINP_CANMsgValidIVI2_flg/1 -> VALUE_TYPE_FlasherSignal/7(VINP_CANMsgValidIVI2_flg)
  VINP_FlashPTGOpenHeight12_enum/1 -> VALUE_TYPE_FlasherSignal/4(EEP_Set12)
  Switch4/1 -> [VBCM_PTGIsSetHeight_flg]
  Switch/1 -> [VBCM_PTGLeftHallPosn_cnt]  "VBCM_PTGLeftHallPosn_cnt"
  VINP_PTGLeftHallPosn_cnt/1 -> Data Type Conversion14/1
  VINP_PTGIsSetHeight_flg/1 -> Switch4/3
  [VINP_CANMsgValidBodyZonePS1_flg] -> Switch/2
  [VINP_CANMsgValidBodyZonePS1_flg] -> Switch4/2
  Switch3/1 -> [VBCM_FlashPTGUserHeight1_cnt]
  [VBCM_PTGDefMaxOpenHeight_cnt] -> Switch3/1
  Compare To Constant1/1 -> Switch3/2
  Data Type Conversion14/1 -> Switch/1
  VINP_BPPTGIsSetHeightSta_flg/1 -> Switch4/1
  [VBCM_FlashPTGUserHeight1_cnt] -> VALUE_TYPE_PTGUserSetMaxHeight/5(EEP_Set1)
  VINP_FlashPTGUserHeight1_cnt/1 -> Switch3/3, Compare To Constant1/1
  [VBCM_PTGLeftHallPosn_cnt] -> VALUE_TYPE_PTGUserSetMaxHeight/4(VINP_PTGLeftHallPosn_cnt)
  [VBCM_PTGIsSetHeight_flg] -> VALUE_TYPE_PTGUserSetMaxHeight/3(VINP_PTGIsSetHeightSta_flg)
  VINP_CANMsgValidBodyZonePS1_flg/1 -> [VINP_CANMsgValidBodyZonePS1_flg]
  Switch1/1 -> Switch/3  "VBCM_PTGLeftHallPosn_cnt"
  OR/1 -> Switch1/2
  Compare To Constant/1 -> OR/1
  VINP_LeftHallPos_cnt/1 -> Data Type Conversion10/1, Compare To Constant2/1, Compare To Constant/1
  Compare To Constant2/1 -> OR/2
  Data Type Conversion9/1 -> Switch1/1
  Data Type Conversion10/1 -> Switch1/3
  Constant9/1 -> Data Type Conversion9/1
  Constant7/1 -> VALUE_TYPE_FlasherSignal/9(Default)
  VINP_VehicleType_enum/1 -> [VINP_VehicleType_enum]
  [VINP_VehicleType_enum] -> Equal/1
  Constant10/1 -> Equal/2
  Equal/1 -> Switch2/2
  Data Type Conversion8/1 -> Switch2/3
  Data Type Conversion7/1 -> Switch2/1
  Constant11/1 -> Data Type Conversion7/1
  Constant12/1 -> Data Type Conversion8/1
  Switch2/1 -> [VBCM_PTGDefMaxOpenHeight_cnt]
  [VBCM_PTGDefMaxOpenHeight_cnt] -> VALUE_TYPE_PTGUserSetMaxHeight/12(Default)

== system bcm/BCM/BCM/Personal_Setting/RoomLamp ==
  UserNow : Inport
  Loadbar : Inport  Port=2
  VINP_RoomLampMode_flg : Inport  Port=3
  VINP_FlashRmLpModeEN_enum : Inport  Port=4
  VINP_SWC2RCustomizeSta_flg : Inport  Port=5
  VINP_IVISWCRUndefinedSta_enum : Inport  Port=6
  HMI_AutoInterLight_Cmd : Inport  Port=7
  AND : Logic  AllPortsSameDT=off  OutDataTypeStr=boolean
  AND1 : Logic  Operator=OR  Inputs=3  AllPortsSameDT=off  OutDataTypeStr=boolean
  Compare To Constant : simulink/Logic and Bit Operations/Compare To Constant  relop===  const=2  OutDataTypeStr=boolean
  Constant : Constant  OutDataTypeStr=boolean
  Detect Increase : simulink/Logic and Bit Operations/Detect Increase  vinit=0.0  OutDataTypeStr=boolean
  Detect Increase1 : simulink/Logic and Bit Operations/Detect Increase  vinit=0.0  OutDataTypeStr=boolean
  Detect Increase2 : simulink/Logic and Bit Operations/Detect Increase  vinit=0.0  OutDataTypeStr=boolean
  TOGGLE_TYPE_RoomLampMode : Subsystem
  FDC_BCM_RmLpModeENFun_Sta : Outport
  VBCM_RmLpModeENMem_enum : Outport  Port=2
  wires:
  TOGGLE_TYPE_RoomLampMode/1(Setting) -> FDC_BCM_RmLpModeENFun_Sta/1
  TOGGLE_TYPE_RoomLampMode/2(Set) -> VBCM_RmLpModeENMem_enum/1
  UserNow/1 -> [UserNow]
  Loadbar/1 -> [Loadbar]
  [UserNow] -> TOGGLE_TYPE_RoomLampMode/1(UserNow)
  [Loadbar] -> TOGGLE_TYPE_RoomLampMode/2(Loadbar)
  VINP_FlashRmLpModeEN_enum/1 -> TOGGLE_TYPE_RoomLampMode/4(EEP_Set)
  Constant/1 -> TOGGLE_TYPE_RoomLampMode/5(Default)
  VINP_IVISWCRUndefinedSta_enum/1 -> Compare To Constant/1
  VINP_SWC2RCustomizeSta_flg/1 -> Detect Increase/1
  HMI_AutoInterLight_Cmd/1 -> Detect Increase1/1
  Detect Increase/1 -> AND/1
  Compare To Constant/1 -> AND/2
  AND1/1 -> TOGGLE_TYPE_RoomLampMode/3(iviCMD)
  AND/1 -> AND1/2
  Detect Increase1/1 -> AND1/3
  VINP_RoomLampMode_flg/1 -> Detect Increase2/1
  Detect Increase2/1 -> AND1/1

== system bcm/BCM/BCM/Personal_Setting/SPTG ==
  UserNow : Inport
  Loadbar : Inport  Port=2
  VINP_IVIPTGUSStaSW_flg : Inport  Port=3
  VINP_FlashSPTGENFun_enum : Inport  Port=4
  Constant1 : Constant  OutDataTypeStr=boolean
  TOGGLE_TYPE_AmbFunEN : Subsystem
  FDC_SPTG_SPTGENFun_Sta : Outport
  VBCM_SPTGENFunMem_enum : Outport  Port=2
  wires:
  UserNow/1 -> TOGGLE_TYPE_AmbFunEN/1(UserNow)
  Loadbar/1 -> TOGGLE_TYPE_AmbFunEN/2(Loadbar)
  VINP_IVIPTGUSStaSW_flg/1 -> TOGGLE_TYPE_AmbFunEN/3(iviCMD)
  VINP_FlashSPTGENFun_enum/1 -> TOGGLE_TYPE_AmbFunEN/4(EEP_Set)
  Constant1/1 -> TOGGLE_TYPE_AmbFunEN/5(Default)
  TOGGLE_TYPE_AmbFunEN/1(Setting) -> FDC_SPTG_SPTGENFun_Sta/1
  TOGGLE_TYPE_AmbFunEN/2(Set) -> VBCM_SPTGENFunMem_enum/1

== system bcm/BCM/BCM/Personal_Setting/System_Loadbar ==
  Add : Sum
  Compare To Constant : simulink/Logic and Bit Operations/Compare To Constant  relop=>  const=2  OutDataTypeStr=boolean
  Constant6 : Constant  Value=0  OutDataTypeStr=uint8
  Constant7 : Constant  OutDataTypeStr=uint8
  Switch7 : Switch  Criteria=u2 > Threshold
  Unit Delay : UnitDelay  SampleTime=-1  HasFrameUpgradeWarning=on
  Unit Delay6 : UnitDelay  SampleTime=-1  HasFrameUpgradeWarning=on
  Loadbar : Outport
  wires:
  Constant7/1 -> Switch7/3
  Unit Delay6/1 -> Add/1
  Switch7/1 -> Add/2
  Unit Delay/1 -> Switch7/2
  Compare To Constant/1 -> Unit Delay/1, Loadbar/1
  Add/1 -> Unit Delay6/1, Compare To Constant/1
  Constant6/1 -> Switch7/1

== system bcm/BCM/BCM/Personal_Setting/Window ==
  UserNow : Inport
  Loadbar : Inport  Port=2
  UpdateReq : Inport  Port=3
  VINP_IVICLWinLockDrSW_flg : Inport  Port=4
  VINP_FlashCLWinLockDrSta_enum : Inport  Port=5
  Constant : Constant  Value=TRUE
  TOGGLE_TYPE_CLWinOWhenLock : $bdroot/BCM/BCM/Personal_Setting/Autolock/TOGGLE_TYPE_AutoLock  SystemSampleTime=-1  VariantActivationTime=update diagram  Latency=0  AutoFrameSizeCalculation=off
  VBCM_CLWinLockDrSta_flg : Outport
  VBCM_CLWinLockDrStaMem_enum : Outport  Port=2
  wires:
  Constant/1 -> TOGGLE_TYPE_CLWinOWhenLock/6
  UserNow/1 -> TOGGLE_TYPE_CLWinOWhenLock/1
  Loadbar/1 -> TOGGLE_TYPE_CLWinOWhenLock/2
  UpdateReq/1 -> TOGGLE_TYPE_CLWinOWhenLock/3
  VINP_IVICLWinLockDrSW_flg/1 -> TOGGLE_TYPE_CLWinOWhenLock/4
  VINP_FlashCLWinLockDrSta_enum/1 -> TOGGLE_TYPE_CLWinOWhenLock/5
  TOGGLE_TYPE_CLWinOWhenLock/1 -> VBCM_CLWinLockDrSta_flg/1  "VBCM_CLWinLockDrSta_flg"
  TOGGLE_TYPE_CLWinOWhenLock/2 -> VBCM_CLWinLockDrStaMem_enum/1  "VBCM_CLWinLockDrStaMem_enum"

== system bcm/BCM/BCM/WasherWiper/RLS_Command_Cut_Filter ==
  VINP_RLSRainSnrWiperCmd_enum : Inport
  task_time_s : Inport  Port=2
  VINP_DiagWipRLSCmdCutEN_flg : Inport  Port=3
  VINP_DiagRLSCmdCutTime_s : Inport  Port=4
  Add : Sum
  Add1 : Sum
  Constant : Constant  Value=2
  Constant1 : Constant  Value=3
  Constant10 : Constant  Value=ONE_INT16
  Constant2 : Constant  Value=ZERO_INT16
  Constant3 : Constant  Value=ONE_INT16
  Constant4 : Constant  Value=3
  Constant5 : Constant  Value=3
  Constant8 : Constant  Value=KBCM_RLSLowSpdFilterT_s
  Constant9 : Constant  Value=ZERO_INT16
  Data Type Conversion : DataTypeConversion  OutDataTypeStr=single
  Data Type Conversion{1..2,5..6} (4 alike) : DataTypeConversion  OutDataTypeStr=uint8
  Data Type Conversion9 : DataTypeConversion  OutDataTypeStr=uint16
  Divide : Product  Inputs=*/
  Divide1 : Product  Inputs=*/
  Equal : RelationalOperator  Operator===  OutDataTypeStr=boolean  RndMeth=Simplest
  Equal1 : RelationalOperator  Operator===  OutDataTypeStr=boolean  RndMeth=Simplest
  Less Than : RelationalOperator  Operator=>  OutDataTypeStr=boolean  RndMeth=Simplest
  OR : Logic  Operator=OR  AllPortsSameDT=off  OutDataTypeStr=boolean
  Relational Operator : RelationalOperator  Operator===  OutDataTypeStr=boolean  RndMeth=Simplest
  Relational Operator1 : RelationalOperator  Operator=>  OutDataTypeStr=boolean  RndMeth=Simplest
  Saturation : Saturate  UpperLimit=1000  LowerLimit=0
  Saturation1 : Saturate  UpperLimit=65500  LowerLimit=0
  Switch : Switch  Criteria=u2 ~= 0
  Switch{1..6} (6 alike) : Switch  Criteria=u2 > Threshold
  Unit Delay{,1..3} (4 alike) : UnitDelay  SampleTime=-1  HasFrameUpgradeWarning=on
  RLS_WiperCmd : Outport
  wires:
  Data Type Conversion5/1 -> Switch3/1
  Unit Delay2/1 -> Switch4/1
  Constant5/1 -> Data Type Conversion5/1
  Switch2/1 -> Saturation/1
  Add/1 -> Switch2/1
  VINP_RLSRainSnrWiperCmd_enum/1 -> [VINP_RLSRainSnrWiperCmd_enum]
  Switch4/1 -> Switch3/3, Unit Delay2/1
  [VINP_RLSRainSnrWiperCmd_enum] -> Switch4/3
  Relational Operator1/1 -> Switch3/2
  Unit Delay1/1 -> Add/1
  Data Type Conversion2/1 -> Relational Operator/2
  [VINP_RLSRainSnrWiperCmd_enum] -> Relational Operator/1
  Constant1/1 -> Data Type Conversion2/1
  Relational Operator/1 -> Switch4/2, Switch2/2
  Saturation/1 -> Relational Operator1/1, Unit Delay1/1
  Divide/1 -> Relational Operator1/2
  VINP_DiagRLSCmdCutTime_s/1 -> Data Type Conversion/1
  VINP_DiagWipRLSCmdCutEN_flg/1 -> Switch/2
  Switch3/1 -> Switch/1
  [VINP_RLSRainSnrWiperCmd_enum] -> Switch/3
  Data Type Conversion/1 -> Divide/1
  [VINP_RLSRainSnrWiperCmd_enum] -> Equal/1
  Constant/1 -> Data Type Conversion1/1
  Data Type Conversion1/1 -> Equal/2
  Data Type Conversion6/1 -> Equal1/2
  Constant4/1 -> Data Type Conversion6/1
  [VINP_RLSRainSnrWiperCmd_enum] -> Equal1/1
  Equal/1 -> OR/1
  Equal1/1 -> OR/2
  OR/1 -> Switch5/2, Switch1/2
  Add1/1 -> Switch1/1
  Unit Delay/1 -> Add1/1
  Switch1/1 -> Saturation1/1
  Saturation1/1 -> Less Than/1, Unit Delay/1
  Switch5/1 -> Unit Delay3/1, Switch6/3
  Unit Delay3/1 -> Switch5/1
  Data Type Conversion9/1 -> Less Than/2
  Less Than/1 -> Switch6/2
  Switch6/1 -> RLS_WiperCmd/1
  Switch/1 -> Switch5/3, Switch6/1
  task_time_s/1 -> [task_time_s]
  [task_time_s] -> Divide/2
  Constant8/1 -> Divide1/1
  [task_time_s] -> Divide1/2
  Divide1/1 -> Data Type Conversion9/1
  Constant10/1 -> Add/2
  Constant9/1 -> Switch2/3
  Constant2/1 -> Switch1/3
  Constant3/1 -> Add1/2
